simulink model "labFinal_5"  (R2018b)
settings: Solver=FixedStepDiscrete  StartTime=0.0  StopTime=10.0  FixedStep=1  RelTol=1e-3
settings Model: Creator=mllax8  LastModifiedBy=mllax8

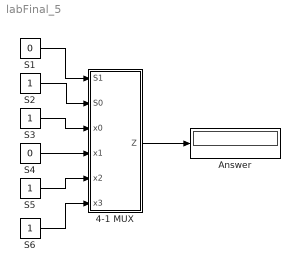
== system labFinal_5 ==
  4-1 MUX : Subsystem
  Answer : Display
  S1 : Constant  Value=0  OutDataTypeStr=uint8  SampleTime=1
  S{2..3,5..6} (4 alike) : Constant  OutDataTypeStr=uint8  SampleTime=1
  S4 : Constant  Value=0  OutDataTypeStr=uint8  SampleTime=1
  wires:
  4-1 MUX/1(Z) -> Answer/1
  S2/1 -> 4-1 MUX/2(S0)
  S1/1 -> 4-1 MUX/1(S1)
  S3/1 -> 4-1 MUX/3(x0)
  S4/1 -> 4-1 MUX/4(x1)
  S5/1 -> 4-1 MUX/5(x2)
  S6/1 -> 4-1 MUX/6(x3)

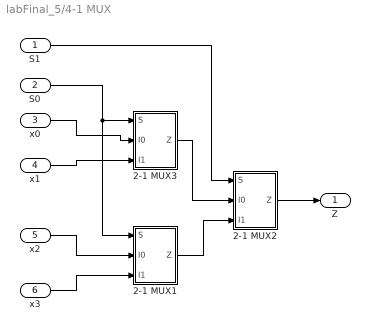
== system labFinal_5/4-1 MUX ==
  S1 : Inport  OutDataTypeStr=uint8
  S0 : Inport  Port=2  OutDataTypeStr=uint8
  x0 : Inport  Port=3  OutDataTypeStr=uint8
  x1 : Inport  Port=4  OutDataTypeStr=uint8
  x2 : Inport  Port=5  OutDataTypeStr=uint8
  x3 : Inport  Port=6  OutDataTypeStr=uint8
  2-1 MUX1 : Subsystem
  2-1 MUX2 : Subsystem
  2-1 MUX3 : Subsystem
  Z : Outport
  wires:
  S0/1 -> 2-1 MUX3/1(S), 2-1 MUX1/1(S)
  x0/1 -> 2-1 MUX3/2(I0)
  x1/1 -> 2-1 MUX3/3(I1)
  x2/1 -> 2-1 MUX1/2(I0)
  x3/1 -> 2-1 MUX1/3(I1)
  2-1 MUX3/1(Z) -> 2-1 MUX2/2(I0)
  2-1 MUX1/1(Z) -> 2-1 MUX2/3(I1)
  S1/1 -> 2-1 MUX2/1(S)
  2-1 MUX2/1(Z) -> Z/1

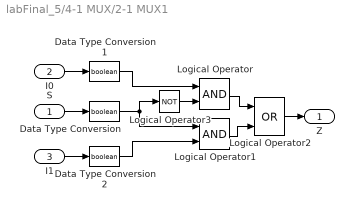
== system labFinal_5/4-1 MUX/2-1 MUX1 ==
  S : Inport  OutDataTypeStr=uint8
  I0 : Inport  Port=2
  I1 : Inport  Port=3
  Data Type Conversion : DataTypeConversion  OutDataTypeStr=boolean
  Data Type Conversion1 : DataTypeConversion  OutDataTypeStr=boolean
  Data Type Conversion2 : DataTypeConversion  OutDataTypeStr=boolean
  Logical Operator : Logic  AllPortsSameDT=off  OutDataTypeStr=boolean
  Logical Operator1 : Logic  AllPortsSameDT=off  OutDataTypeStr=boolean
  Logical Operator2 : Logic  Operator=OR  AllPortsSameDT=off  OutDataTypeStr=boolean
  Logical Operator3 : Logic  Operator=NOT  AllPortsSameDT=off  OutDataTypeStr=boolean
  Z : Outport
  wires:
  Logical Operator2/1 -> Z/1
  I1/1 -> Data Type Conversion2/1
  Logical Operator1/1 -> Logical Operator2/2
  Data Type Conversion/1 -> Logical Operator3/1, Logical Operator1/1
  I0/1 -> Data Type Conversion1/1
  Logical Operator/1 -> Logical Operator2/1
  S/1 -> Data Type Conversion/1
  Data Type Conversion1/1 -> Logical Operator/1
  Data Type Conversion2/1 -> Logical Operator1/2
  Logical Operator3/1 -> Logical Operator/2

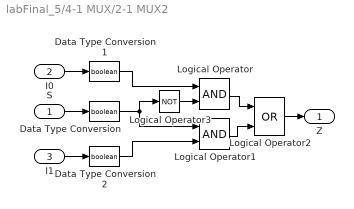
== system labFinal_5/4-1 MUX/2-1 MUX2 ==
  S : Inport  OutDataTypeStr=uint8
  I0 : Inport  Port=2
  I1 : Inport  Port=3
  Data Type Conversion : DataTypeConversion  OutDataTypeStr=boolean
  Data Type Conversion1 : DataTypeConversion  OutDataTypeStr=boolean
  Data Type Conversion2 : DataTypeConversion  OutDataTypeStr=boolean
  Logical Operator : Logic  AllPortsSameDT=off  OutDataTypeStr=boolean
  Logical Operator1 : Logic  AllPortsSameDT=off  OutDataTypeStr=boolean
  Logical Operator2 : Logic  Operator=OR  AllPortsSameDT=off  OutDataTypeStr=boolean
  Logical Operator3 : Logic  Operator=NOT  AllPortsSameDT=off  OutDataTypeStr=boolean
  Z : Outport
  wires:
  Logical Operator2/1 -> Z/1
  I1/1 -> Data Type Conversion2/1
  Logical Operator1/1 -> Logical Operator2/2
  Data Type Conversion/1 -> Logical Operator3/1, Logical Operator1/1
  I0/1 -> Data Type Conversion1/1
  Logical Operator/1 -> Logical Operator2/1
  S/1 -> Data Type Conversion/1
  Data Type Conversion1/1 -> Logical Operator/1
  Data Type Conversion2/1 -> Logical Operator1/2
  Logical Operator3/1 -> Logical Operator/2

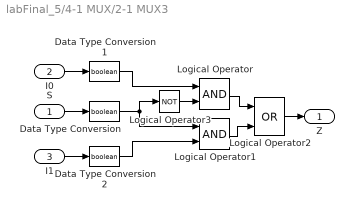
== system labFinal_5/4-1 MUX/2-1 MUX3 ==
  S : Inport  OutDataTypeStr=uint8
  I0 : Inport  Port=2
  I1 : Inport  Port=3
  Data Type Conversion : DataTypeConversion  OutDataTypeStr=boolean
  Data Type Conversion1 : DataTypeConversion  OutDataTypeStr=boolean
  Data Type Conversion2 : DataTypeConversion  OutDataTypeStr=boolean
  Logical Operator : Logic  AllPortsSameDT=off  OutDataTypeStr=boolean
  Logical Operator1 : Logic  AllPortsSameDT=off  OutDataTypeStr=boolean
  Logical Operator2 : Logic  Operator=OR  AllPortsSameDT=off  OutDataTypeStr=boolean
  Logical Operator3 : Logic  Operator=NOT  AllPortsSameDT=off  OutDataTypeStr=boolean
  Z : Outport
  wires:
  Logical Operator2/1 -> Z/1
  I1/1 -> Data Type Conversion2/1
  Logical Operator1/1 -> Logical Operator2/2
  Data Type Conversion/1 -> Logical Operator3/1, Logical Operator1/1
  I0/1 -> Data Type Conversion1/1
  Logical Operator/1 -> Logical Operator2/1
  S/1 -> Data Type Conversion/1
  Data Type Conversion1/1 -> Logical Operator/1
  Data Type Conversion2/1 -> Logical Operator1/2
  Logical Operator3/1 -> Logical Operator/2
